simulink model "test"  (R2017a)
settings: Solver=VariableStepAuto  StartTime=0.0  StopTime=500  RelTol=1e-3
values from neighbouring files (symbols this model uses):
  K_pd = (sqrt(w_c.^4*T_f.^2+w_c.^2))./K    [p5p5a.m]    (also in p5p5c.m; p5p5d.m; p5p5e.m)
  T_d = T    (= 72.4357)    [p5p5a.m]    (also in p5p5c.m; p5p5d.m; p5p5e.m)
  T_f = 1/(w_c*tan(-130*pi/180))    [p5p5a.m]    (also in p5p5c.m; p5p5d.m; p5p5e.m)
  Ts = 0.1    [p5p5a.m]    (also in p5p5c.m; p5p5d.m; p5p5e.m)
  w_r = 30    [p5p5a.m]    (also in p5p5c.m; p5p5d.m; p5p5e.m)
libraries: simulink_extras x6, simulink x2
settings Model: Creator=Toragh  LastModifiedBy=Toragh

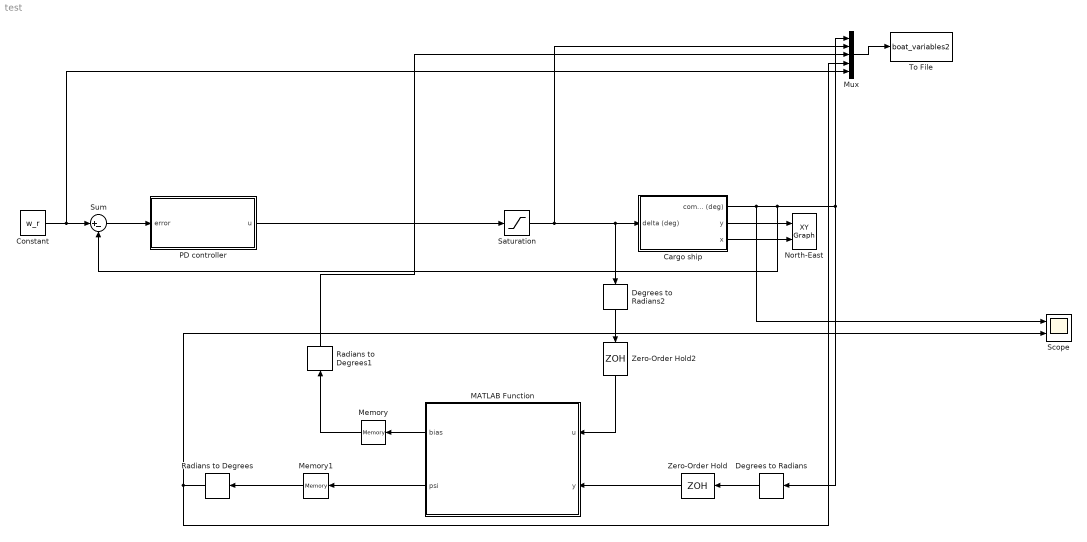
== system test ==
  Cargo ship : Subsystem  mask(Simple shipmodel for a cargo ship){noise=on, current=on, logic=on}
      mask prompts: noise "measurement noise"; logic "waves"
      mask help:
      | Measurement noise:
      | 	checked = noise on
      | 	unchecked = noise off
      |
      | Current:
      | 	checked = current on
      | 	unchecked = current off
      |
      | Waves:
      | 	checked = waves on
      | 	unchecked = waves off
      |
      | Author: Jørgen Spjøtvold, 9/10-2003
      | TTK 4115 Linear system theory.
      | Modified by Jostein Bakkeheim 26/10-2006
  Constant : Constant  Value=w_r
  Degrees to Radians : simulink_extras/Transformations/Degrees to Radians
  Degrees to Radians2 : simulink_extras/Transformations/Degrees to Radians
  MATLAB Function : MATLAB Function  TreatAsAtomicUnit=on
  Memory : Memory
  Memory1 : Memory
  Mux : Mux  Inputs=5
  North-East : simulink/Sinks/XY Graph  xmin=-5000  xmax=5000  ymin=-5000  ymax=5000  st=-1
  "PD controller " : Subsystem
  Radians to Degrees : simulink_extras/Transformations/Radians to Degrees
  Radians to Degrees1 : simulink_extras/Transformations/Radians to Degrees
  Saturation : Saturate  UpperLimit=35  LowerLimit=-35
  Scope : Scope  NumInputPorts=2
  Sum : Sum  Inputs=|+-
  To File : ToFile  Filename=boat_variables2
  Zero-Order Hold : ZeroOrderHold  SampleTime=Ts
  Zero-Order Hold2 : ZeroOrderHold  SampleTime=Ts
  wires:
  MATLAB Function/2(psi) -> Memory1/1
  Degrees to Radians2/1 -> Zero-Order Hold2/1
  Memory1/1 -> Radians to Degrees/1
  Constant/1 -> Mux/5, Sum/1
  "PD controller "/1(u) -> Saturation/1
  Zero-Order Hold/1 -> MATLAB Function/2(y)
  Memory/1 -> Radians to Degrees1/1
  Sum/1 -> "PD controller "/1(error)
  Radians to Degrees1/1 -> Mux/3
  Zero-Order Hold2/1 -> MATLAB Function/1(u)
  Degrees to Radians/1 -> Zero-Order Hold/1
  Mux/1 -> To File/1
  Radians to Degrees/1 -> Scope/2, Mux/4
  MATLAB Function/1(bias) -> Memory/1
  Cargo ship/2(y) -> North-East/1
  Cargo ship/3(x) -> North-East/2
  Cargo ship/1(compass (deg)) -> Scope/1, Sum/2, Degrees to Radians/1, Mux/1
  Saturation/1 -> Mux/2, Cargo ship/1(delta (deg)), Degrees to Radians2/1

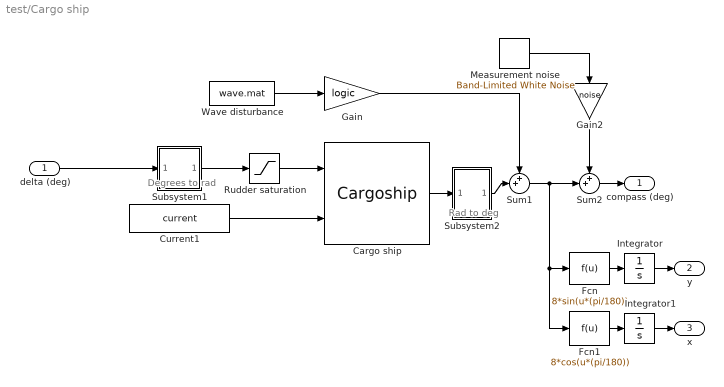
== system test/Cargo ship ==
  note: Degrees to rad
  note: Rad to deg
  delta (deg) : Inport
  Cargo ship : S-Function  FunctionName=Cargoship  SFunctionDeploymentMode=off  EnableBusSupport=off  mask(Cargo ship){}
      mask help:
      | S-function which simulates a cargo ship.
      |
      | Author: Jørgen Spjøtvold
      | 20.10-2003
      | Modified by Jostein Bakkeheim 27.10.2006
  Current1 : Constant  Value=current
  Fcn : Fcn  Expr=8*sin(u*(pi/180))
  Fcn1 : Fcn  Expr=8*cos(u*(pi/180))
  Gain : Gain  Gain=logic  SaturateOnIntegerOverflow=on  OutDataTypeStr=Inherit: Same as input  ParamDataTypeStr=Inherit: Same as input
  Gain2 : Gain  Gain=noise  SaturateOnIntegerOverflow=on  OutDataTypeStr=Inherit: Same as input  ParamDataTypeStr=Inherit: Same as input
  Integrator : Integrator
  Integrator1 : Integrator
  Measurement noise : simulink/Sources/Band-Limited White Noise  Cov=[0.001]  Ts=.5  seed=[23341]
  Rudder saturation : Saturate  UpperLimit=45*(pi/180)  LowerLimit=-45*(pi/180)
  Subsystem1 : Subsystem  mask(degrees to radians){}
      mask help: Converts degrees to radians
      mask Display: fprintf('D2R');
  Subsystem2 : Subsystem  mask(radians to degrees){}
      mask help: Converts radians to degrees
      mask Display: fprintf('R2D');
  Sum1 : Sum  Inputs=++|  SaturateOnIntegerOverflow=on
  Sum2 : Sum  Inputs=++|  SaturateOnIntegerOverflow=on
  Wave disturbance : FromFile  FileName=wave.mat  SampleTime=0
  compass (deg) : Outport
  y : Outport  Port=2
  x : Outport  Port=3
  wires:
  delta (deg)/1 -> Subsystem1/1(In1)
  Fcn/1 -> Integrator/1
  Integrator/1 -> y/1
  Fcn1/1 -> Integrator1/1
  Integrator1/1 -> x/1
  Wave disturbance/1 -> Gain/1
  Subsystem2/1(Out1) -> Sum1/2
  Gain/1 -> Sum1/1
  Sum1/1 -> Fcn/1, Fcn1/1, Sum2/2
  Cargo ship/1 -> Subsystem2/1(In1)
  Subsystem1/1(Out1) -> Rudder saturation/1
  Rudder saturation/1 -> Cargo ship/1
  Sum2/1 -> compass (deg)/1
  Measurement noise/1 -> Gain2/1
  Gain2/1 -> Sum2/1
  Current1/1 -> Cargo ship/2

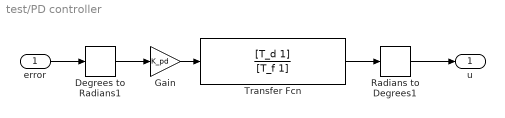
== system test/PD controller  ==
  error : Inport
  Degrees to Radians1 : simulink_extras/Transformations/Degrees to Radians
  Gain : Gain  Gain=K_pd
  Radians to Degrees1 : simulink_extras/Transformations/Radians to Degrees
  Transfer Fcn : TransferFcn  Numerator=[T_d 1]  Denominator=[T_f 1]
  u : Outport
  wires:
  Radians to Degrees1/1 -> u/1
  Degrees to Radians1/1 -> Gain/1
  Gain/1 -> Transfer Fcn/1
  Transfer Fcn/1 -> Radians to Degrees1/1
  error/1 -> Degrees to Radians1/1

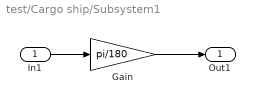
== system test/Cargo ship/Subsystem1 ==
  In1 : Inport
  Gain : Gain  Gain=pi/180  SaturateOnIntegerOverflow=on  OutDataTypeStr=Inherit: Same as input  ParamDataTypeStr=Inherit: Same as input
  Out1 : Outport
  wires:
  Gain/1 -> Out1/1
  In1/1 -> Gain/1

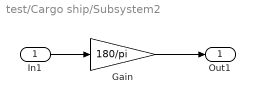
== system test/Cargo ship/Subsystem2 ==
  In1 : Inport
  Gain : Gain  Gain=180/pi  SaturateOnIntegerOverflow=on  OutDataTypeStr=Inherit: Same as input  ParamDataTypeStr=Inherit: Same as input
  Out1 : Outport
  wires:
  Gain/1 -> Out1/1
  In1/1 -> Gain/1

== matlab function test/MATLAB Function ==
  data: u input; bias output; psi output; y input
function [bias, psi] = kalman_f(u, y)
    persistent init_flag x_pri P_pri
    P_pri_0 = [1 0 0 0 0;0 0.013 0 0 0; 0 0 pi^2 0 0; 0 0 0 1 0;0 0 0 0 2.5*10^-3];
    x_pri_0 = [0; 0; 0; 0; 0];
    Q = [30 0; 0 1e-06];
    R = 6.051993621726547e-06;
    I =diag([1 1 1 1 1]);
    
    Ad = [0.996954741048002 0.0992545087604663 0 0 0;
        -0.0607430933636516 0.984111959963574 0 0 0;
        0 0 1 0.0999310050168264 -1.07701168734005e-05;
        0 0 0 0.998620417763384 -0.000215352787135716;
        0 0 0 0 1];
    Bd = [0;0;1.07701168734005e-05;0.000215352787135716;0];
    Cd = [0 1 1 0 0];
    Ed = [1.811858664137177e-05 0;
        3.614073605307908e-04 0;
        0 -3.590451934240905e-07;
        0 -1.077011687340049e-05;
        0 0.100000000000000];
    
    if (isempty(init_flag))
        init_flag = 1;
        P_pri = P_pri_0;
        x_pri = x_pri_0;
    end
        K = (P_pri*Cd.')*(inv(Cd*P_pri*Cd.'+R));
        x = x_pri + K*(y-Cd*x_pri); 
        P = (I-K*Cd)*P_pri*(I-K*Cd).'+K*R*K.';
        
        x_pri = Ad*x + Bd*u;
        P_pri = Ad*P*(Ad.') + Ed*Q*(Ed.');
        
        psi = x(3);
        bias = x(5);
end
